simulink model "Act_2"  (R2024a)
settings: Solver=VariableStepAuto  StartTime=0.0  StopTime=10.0  RelTol=1e-3
settings Model: Creator=ansm3  LastModifiedBy=ansm3

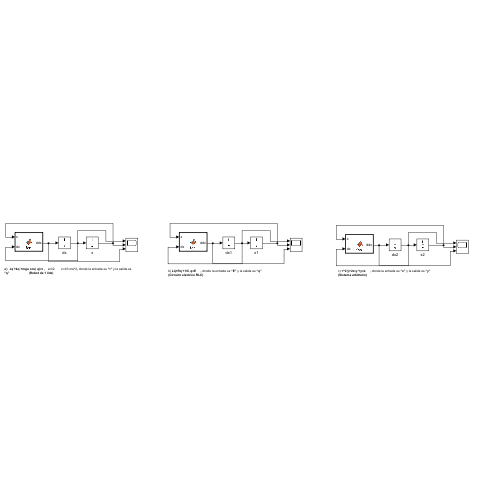
[thumbnail: Simulink's stored preview of the top-level diagram]
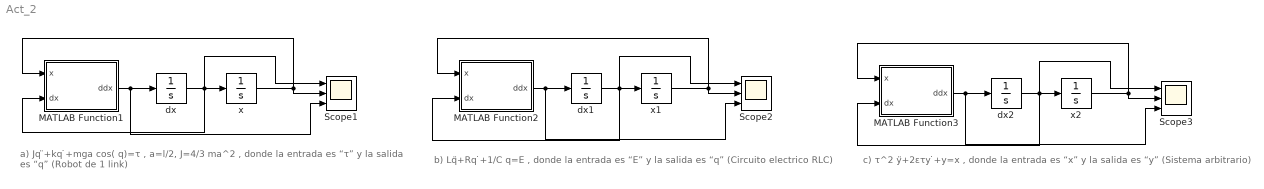
== system Act_2 ==
  note: a) Jq ̈+kq ̇+mga cos⁡( q)=τ , a=l/2, J=4/3 ma^2 , donde la entrada es “τ” y la salida es “q” (Robot de 1 link)
  note: b) Lq̈+Rq ̇+1/C q=E , donde la entrada es “E” y la salida es “q” (Circuito electrico RLC)
  note: c) τ^2 ÿ+2ετy ̇+y=x , donde la entrada es “x” y la salida es “y” (Sistema arbitrario)
  MATLAB Function1 : MATLAB Function  TreatAsAtomicUnit=on
  MATLAB Function2 : MATLAB Function  TreatAsAtomicUnit=on
  MATLAB Function3 : MATLAB Function  TreatAsAtomicUnit=on
  Scope1 : Scope  NumInputPorts=3
  Scope2 : Scope  NumInputPorts=3
  Scope3 : Scope  NumInputPorts=3
  dx : Integrator  ContinuousStateAttributes="\"dx\""
  dx1 : Integrator  ContinuousStateAttributes="\"dx\""
  dx2 : Integrator  ContinuousStateAttributes="\"dx\""
  x : Integrator
  x1 : Integrator
  x2 : Integrator
  wires:
  MATLAB Function2/1(ddx) -> Scope2/3, dx1/1
  dx1/1 -> Scope2/1, MATLAB Function2/2(dx), x1/1
  x1/1 -> Scope2/2, MATLAB Function2/1(x)
  MATLAB Function3/1(ddx) -> Scope3/3, dx2/1
  dx2/1 -> Scope3/1, MATLAB Function3/2(dx), x2/1
  x2/1 -> Scope3/2, MATLAB Function3/1(x)
  MATLAB Function1/1(ddx) -> Scope1/3, dx/1
  x/1 -> Scope1/2, MATLAB Function1/1(x)
  dx/1 -> Scope1/1, MATLAB Function1/2(dx), x/1

== matlab function Act_2/MATLAB Function2 ==
  data: x input; ddx output; dx input
function ddx = fcn(x, dx)

ddx=(1/L*C)-((R/L)*dx)+E/L;

== matlab function Act_2/MATLAB Function3 ==
  data: x input; ddx output; dx input
function ddx = fcn(x, dx)

ddx=(x/tao^2)-((2*Edx2)/tao)-(x1/tao^2);

== matlab function Act_2/MATLAB Function1 ==
  data: x input; ddx output; dx input
function ddx = fcn(x, dx)

ddx=(1/J)*(tao-m*g*a*(cos(x1))-k*x2);
